simulink model "KukaForwardTransformationMatrix"  (R2017a)
settings: Solver=VariableStepAuto  StartTime=0.0  StopTime=10.0  RelTol=1e-3
settings Model: Creator=abhishek  LastModifiedBy=abhishek

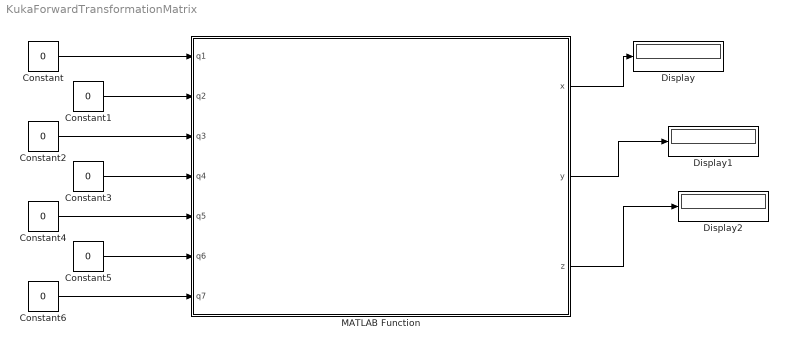
== system KukaForwardTransformationMatrix ==
  Constant{,1..6} (7 alike) : Constant  Value=0
  Display : Display
  Display1 : Display
  Display2 : Display
  MATLAB Function : MATLAB Function  TreatAsAtomicUnit=on
  wires:
  Constant/1 -> MATLAB Function/1(q1)
  MATLAB Function/1(x) -> Display/1
  MATLAB Function/2(y) -> Display1/1
  MATLAB Function/3(z) -> Display2/1
  Constant1/1 -> MATLAB Function/2(q2)
  Constant3/1 -> MATLAB Function/4(q4)
  Constant2/1 -> MATLAB Function/3(q3)
  Constant4/1 -> MATLAB Function/5(q5)
  Constant5/1 -> MATLAB Function/6(q6)
  Constant6/1 -> MATLAB Function/7(q7)

== matlab function KukaForwardTransformationMatrix/MATLAB Function ==
  data: x output; q1 input; y output; q2 input; q3 input; q4 input; q5 input; q6 input; q7 input; z output
function [x,y,z] = fcn(q1,q2,q3,q4,q5,q6,q7)
T1 = [cos(q1),0,sin(q1),0;sin(q1),0,(-1)*cos(q1),0;0,1,0,0.34E0;0,0,0, ...
1];
T2 = [cos(q2),0,(-1)*sin(q2),0;sin(q2),0,cos(q2),0;0,(-1),0,0;0,0,0, ...
  1];
T3 = [cos(q3),0,(-1)*sin(q3),0;sin(q3),0,cos(q3),0;0,(-1),0,0.4E0;0,0, ...
  0,1];
T4 = [cos(q4),0,sin(q4),0;sin(q4),0,(-1)*cos(q4),0;0,1,0,0;0,0,0,1];
T5 = [cos(q5),0,sin(q5),0;sin(q5),0,(-1)*cos(q5),0;0,1,0,0.4E0;0,0,0, ...
  1];
T6 = [cos(q6),0,(-1)*sin(q6),0;sin(q6),0,cos(q6),0;0,(-1),0,0;0,0,0, ...
  1];
T7 = [cos(q7),0,sin(q7),0;sin(q7),0,(-1)*cos(q7),0;0,1,0,0.126E0;0,0, ...
  0,1];

T = T1*T2*T3*T4*T5*T6*T7;

x=T(1,4);
y=T(2,4);
z=T(3,4);
